simulink model "inf_tfl_sim"  (R2024b)
settings: Solver=FixedStepDiscrete  StartTime=0.0  StopTime=10.0  RelTol=1e-3
values from neighbouring files (symbols this model uses):
  input_values = reshape(input(index,:), [dim_1, dim_2])'    [main.m]
  temp_max = 184.88    [main.m]
  temp_min = 19.6    [main.m]
undefined symbols (not defined in the file or in its folder): inf_tfl_mat
settings Model: Creator=dx5entre  LastModifiedBy=dx5entre
settings OptimizationCC: DefaultParameterBehavior=Inlined  UseDivisionForNetSlopeComputation=on  GainParamInheritBuiltInType=on  UseFloatMulNetSlope=on  InlineInvariantSignals=on  EnhancedBackFolding=on  PassReuseOutputArgsThreshold=0  ZeroExternalMemoryAtStartup=off  ZeroInternalMemoryAtStartup=off  EfficientFloat2IntCast=on  OptimizeBlockOrder=speed  DifferentSizesBufferReuse=on  OptimizationCustomize=off
settings DebuggingCC: ParameterTunabilityLossMsg=error
settings SFSimCC: MATLABDynamicMemAlloc=off  SimTargetLang=C++
settings RTWCC: GenCodeOnly=on  Toolchain=CMake  TargetLang=C++
settings CodeAppCC: ForceParamTrailComments=on  OperatorAnnotations=on
settings GRTTargetCC: TargetLangStandard=C++20 (ISO)  CodeInterfacePackaging=C++ class

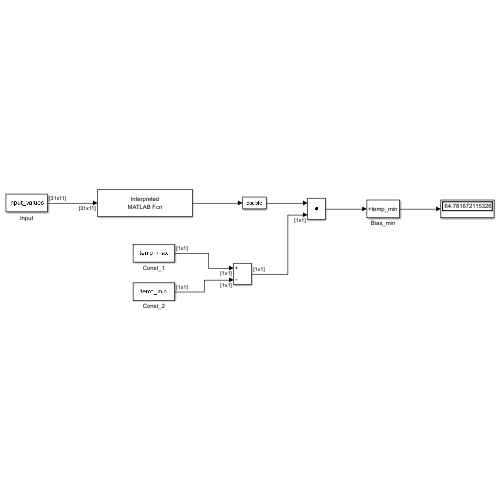
[thumbnail: Simulink's stored preview of the top-level diagram]
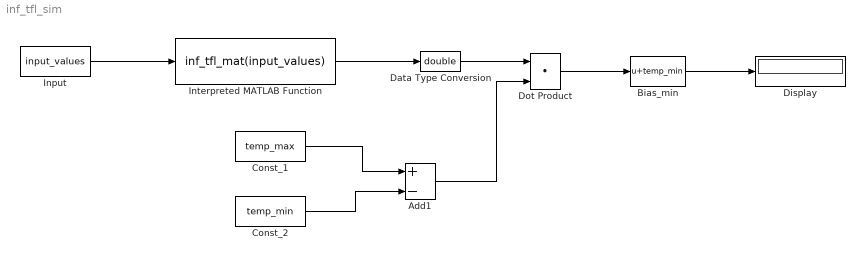
== system inf_tfl_sim ==
  Add1 : Sum  Inputs=+-
  Bias_min : Bias  Bias=temp_min  SaturateOnIntegerOverflow=off
  Const_1 : Constant  Value=temp_max  VectorParams1D=off
  Const_2 : Constant  Value=temp_min  VectorParams1D=off
  Data Type Conversion : DataTypeConversion  OutDataTypeStr=double  SaturateOnIntegerOverflow=off  RndMeth=Floor
  Display : Display
  Dot Product : DotProduct  OutDataTypeStr=Inherit: Inherit via internal rule
  Input : Constant  Value=input_values  VectorParams1D=off
  Interpreted MATLAB Function : MATLABFcn  MATLABFcn=inf_tfl_mat(input_values)  OutputDimensions=1  OutputSignalType=real  Output1D=off
  wires:
  Add1/1 -> Dot Product/2
  Const_2/1 -> Add1/2
  Dot Product/1 -> Bias_min/1
  Input/1 -> Interpreted MATLAB Function/1
  Data Type Conversion/1 -> Dot Product/1
  Interpreted MATLAB Function/1 -> Data Type Conversion/1
  Bias_min/1 -> Display/1
  Const_1/1 -> Add1/1
